simulink model "L_sys"  (R2019b)
settings: Solver=VariableStepAuto  StartTime=0.0  StopTime=20  RelTol=1e-3
undefined symbols (not defined in the file): A_Obs, B_Obs, C_Obs, D_Obs, g, J, K, l, m, Mcart, Noise, Observer
libraries: simulink x1
settings Model: Creator=huojiaxi  LastModifiedBy=huojiaxi
settings DebuggingCC: AlgebraicLoopMsg=none

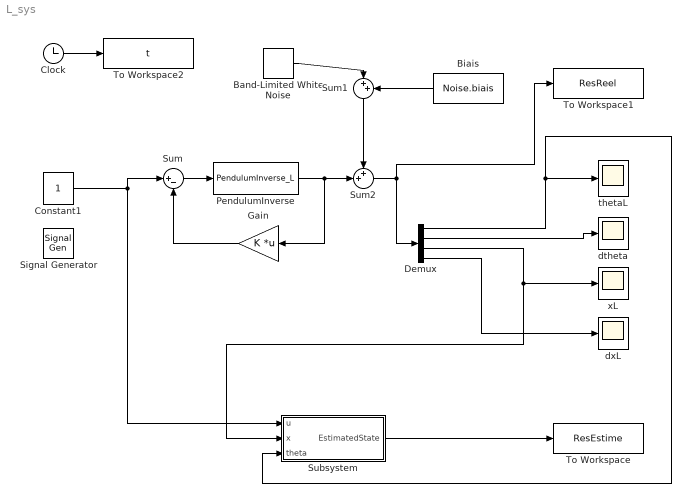
== system L_sys ==
  Band-Limited White Noise : simulink/Sources/Band-Limited White Noise  Cov=Noise.power  Ts=Noise.sampling  seed=Noise.seed
  Biais : Constant  Value=Noise.biais
  Clock : Clock
  Constant1 : Constant
  Demux : Demux
  Gain : Gain  Gain=K  Multiplication=Matrix(K*u) (u vector)
  PendulumInverse : S-Function  FunctionName=PendulumInverse_L  Parameters=Mcart,m,l,g,J  SFunctionDeploymentMode=off  EnableBusSupport=off
  Signal Generator : SignalGenerator  Units=rad/sec
  Subsystem : Subsystem
  Sum : Sum  Inputs=|+-
  Sum1 : Sum  Inputs=|++
  Sum2 : Sum  Inputs=++|
  To Workspace : ToWorkspace  VariableName=ResEstime  SampleTime=-1
  To Workspace1 : ToWorkspace  VariableName=ResReel  SampleTime=-1
  To Workspace2 : ToWorkspace  VariableName=t  SaveFormat=Timeseries  SampleTime=-1
  dtheta : Scope
  "dxL " : Scope
  thetaL : Scope
  xL : Scope
  wires:
  Demux/1 -> Subsystem/3(theta), thetaL/1
  Constant1/1 -> Sum/1, Subsystem/1(u)
  Demux/3 -> xL/1, Subsystem/2("x ")
  Demux/4 -> "dxL "/1
  Demux/2 -> dtheta/1
  Sum/1 -> PendulumInverse/1
  Gain/1 -> Sum/2
  Subsystem/1(EstimatedState) -> To Workspace/1
  PendulumInverse/1 -> Gain/1, Sum2/2
  Clock/1 -> To Workspace2/1
  Band-Limited White Noise/1 -> Sum1/1
  Biais/1 -> Sum1/2
  Sum1/1 -> Sum2/1
  Sum2/1 -> Demux/1, To Workspace1/1

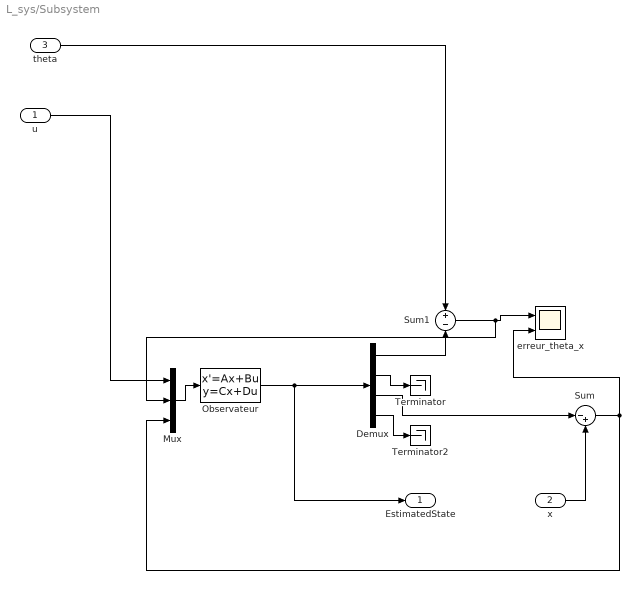
== system L_sys/Subsystem ==
  u : Inport
  "x " : Inport  Port=2
  theta : Inport  Port=3
  Demux : Demux
  Mux : Mux  Inputs=3
  Observateur : StateSpace  A=A_Obs  B=B_Obs  C=C_Obs  D=D_Obs  InitialCondition=Observer.IC
  Sum : Sum  Inputs=|-+
  Sum1 : Sum  Inputs=+-
  Terminator : Terminator
  Terminator2 : Terminator
  erreur_theta_x : Scope  NumInputPorts=2
  EstimatedState : Outport  VectorParamsAs1DForOutWhenUnconnected=off
  wires:
  Demux/3 -> Sum/1
  Demux/2 -> Terminator/1
  Mux/1 -> Observateur/1
  theta/1 -> Sum1/1
  Demux/1 -> Sum1/2
  u/1 -> Mux/1
  Sum1/1 -> Mux/2, erreur_theta_x/1
  Observateur/1 -> EstimatedState/1, Demux/1
  Demux/4 -> Terminator2/1
  "x "/1 -> Sum/2
  Sum/1 -> erreur_theta_x/2, Mux/3
